simulink model "Lab2te"  (R2017b)
settings: Solver=VariableStepAuto  StartTime=0.0  StopTime=200  MaxStep=0.1  RelTol=1e-3
values from neighbouring files (symbols this model uses):
  J = 30    [Labdata.m]
  kdmp = 1.5    [Labdata.m]    (also in lab2_data.m = 2)
  ksp = 12    [Labdata.m]    (also in lab2_data.m = 20)
  M = 10    [Labdata.m]    (also in lab2_data.m = 250)
  wt = abs(imag(wt(1)))    [Labdata.m]
libraries: fl_lib x6, nesl_utility x4
settings Model: Creator=Aleksandr  LastModifiedBy=Aleksandr

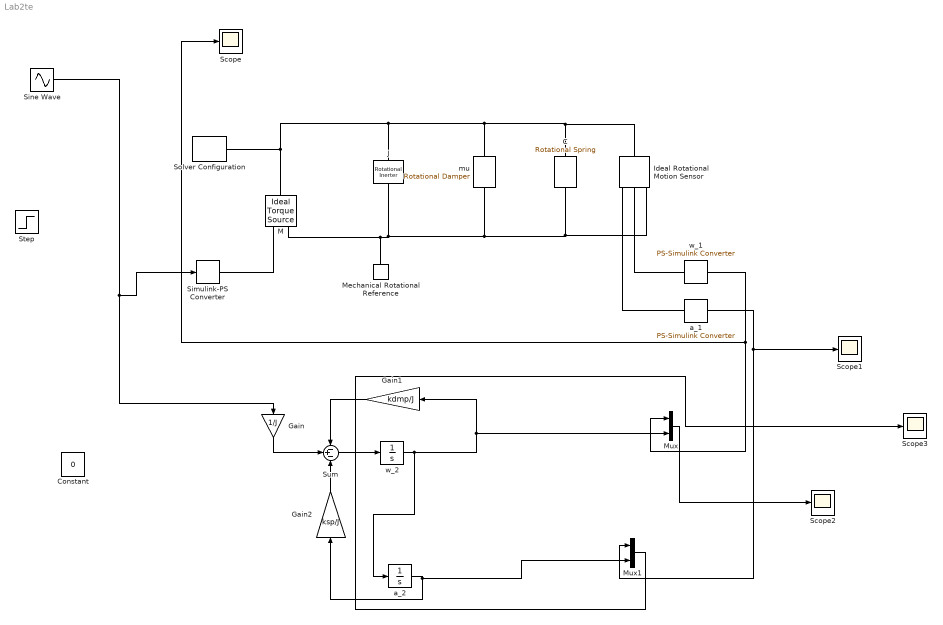
== system Lab2te ==
  C : fl_lib/Mechanical/Rotational Elements/Rotational Spring  spr_rate=ksp N*m/rad  w_specify=off  w_priority=None  w=0 rad/s  w_nominal_specify=off  w_nominal_unit=rad/s  w_nominal_value=1  t_specify=off  t_priority=None  t=0 N*m  t_nominal_specify=off  t_nominal_unit=N*m  t_nominal_value=1  phi_specify=off  phi_priority=High  phi=2 rad  phi_nominal_specify=off  phi_nominal_unit=rad  phi_nominal_value=1
      settings: SourceProductName=Simscape
  Constant : Constant  Value=0
  Gain : Gain  Gain=1/J
  Gain1 : Gain  Gain=kdmp/J
  Gain2 : Gain  Gain=ksp/J
  Ideal Rotational Motion Sensor : fl_lib/Mechanical/Mechanical Sensors/Ideal Rotational Motion Sensor  offset=0 rad
  J : fl_lib/Mechanical/Rotational Elements/Rotational Inerter  B=J kg*m^2  w_specify=off  w_priority=High  w=0 rad/s  w_nominal_specify=off  w_nominal_unit=rad/s  w_nominal_value=1  t_specify=off  t_priority=None  t=0 N*m  t_nominal_specify=off  t_nominal_unit=N*m  t_nominal_value=1
      settings: SourceProductName=Simscape  SourceProductBaseCode=SS
  M : fl_lib/Mechanical/Mechanical Sources/Ideal Torque Source
  Mechanical Rotational Reference : fl_lib/Mechanical/Rotational Elements/Mechanical Rotational Reference
  Mux : Mux  Inputs=2
  Mux1 : Mux  Inputs=2
  Scope{,1..3} (4 alike) : Scope
  Simulink-PS Converter : nesl_utility/Simulink-PS Converter  PhysicalDomain=network_engine_domain  SubClassName=ps_input  LeftPortType=input  RightPortType=output  PseudoPeriodic=off  Frequencies=[]  NoiseDistribution=none  NoiseParameters=[]  Unit=1  AffineConversion=off  FilteringAndDerivatives=provide  SimscapeFilterOrder=1  InputFilterTimeConstant=0.001  UdotUserProvided=0
  Sine Wave : Sin  Amplitude=30  Frequency=wt  SampleTime=0
  Solver Configuration : nesl_utility/Solver Configuration  PhysicalDomain=network_engine_domain  SubClassName=solver  LeftPortType=input  RightPortType=generic  Accelerate=off  Tones=[]  Harmonics=[]  SimulateNoise=off  Profile=off  UseLocalSampling=off  EnableSwitchedLinearOptims=on  FrequencyDomain=off  UseCCode=off  RelTol=0.001  AbsTol=1e-06  MinStep=1e-09  ToWorkspace=off  RevertToSquareIcSolve=off  NumHomotopyIterations=100  PhasorMode=off  PhasorModeNumHarmonics=1  DoDC=off  ResidualTolerance=1e-09  UseLocalSolver=off  LocalSolverChoice=NE_BACKWARD_EULER_ADVANCER  LocalSolverSampleTime=0.001  DoFixedCost=off  MaxNonlinIter=3  MaxModeIter=2  LinearAlgebra=Sparse  DelaysMemoryBudget=1024  AutomaticFiltering=on  FilteringTimeConstant=0.001
  Step : Step  After=M  SampleTime=0
  Sum : Sum  Inputs=-+-
  a_1 : nesl_utility/PS-Simulink Converter  PhysicalDomain=network_engine_domain  SubClassName=ps_output  LeftPortType=input  RightPortType=output  PseudoPeriodic=off  Frequencies=[]  Unit=1  AffineConversion=off
  a_2 : Integrator
  mu : fl_lib/Mechanical/Rotational Elements/Rotational Damper  D=kdmp N*m/(rad/s)  w_specify=off  w_priority=None  w=0 rad/s  w_nominal_specify=off  w_nominal_unit=rad/s  w_nominal_value=1  t_specify=off  t_priority=None  t=0 N*m  t_nominal_specify=off  t_nominal_unit=N*m  t_nominal_value=1
  w_1 : nesl_utility/PS-Simulink Converter  PhysicalDomain=network_engine_domain  SubClassName=ps_output  LeftPortType=input  RightPortType=output  PseudoPeriodic=off  Frequencies=[]  Unit=1  AffineConversion=off
  w_2 : Integrator
  wires:
  w_1/1 -> Mux/1, Scope/1
  a_1/1 -> Mux1/1, Scope1/1
  Sum/1 -> w_2/1
  w_2/1 -> a_2/1, Mux/2, Gain1/1
  Gain1/1 -> Sum/1
  a_2/1 -> Mux1/2, Gain2/1
  Gain2/1 -> Sum/3
  Gain/1 -> Sum/2
  Mux/1 -> Scope2/1
  Mux1/1 -> Scope3/1
  Sine Wave/1 -> Gain/1, Simulink-PS Converter/1
  connections:
  Mechanical Rotational Reference/LConn1 -- Ideal Rotational Motion Sensor/RConn1 -- C/RConn1 -- mu/RConn1 -- J/RConn1 -- M/RConn2
  M/LConn1 -- Solver Configuration/RConn1 -- Ideal Rotational Motion Sensor/LConn1 -- C/LConn1 -- mu/LConn1 -- J/LConn1
  Simulink-PS Converter/RConn1 -- M/RConn1
  Ideal Rotational Motion Sensor/RConn2 -- w_1/LConn1
  Ideal Rotational Motion Sensor/RConn3 -- a_1/LConn1
